simulink model "chase_1"  (R2017b)
settings: Solver=VariableStepAuto  StartTime=0.0  StopTime=400  FixedStep=0.0000001  RelTol=1e-3
values from neighbouring files (symbols this model uses):
  Cwy1 = 0.0074    [Parameters (2).m]    (also in Parameters.m)
  Cwy2 = 0.0527    [Parameters (2).m]    (also in Parameters.m)
  Cx = 52.92    [Parameters (2).m]    (also in Parameters.m)
  Jyy = 0.78    [Parameters (2).m]    (also in Parameters.m)
  k1_k = 0.3    [Parameters (2).m]    (also in Parameters.m)
  k2_k = 0.16732    [Parameters (2).m]    (also in Parameters.m)
  k2_m = 2.19    [Parameters (2).m]    (also in Parameters.m)
  K_thruster = 2.89    [Parameters (2).m]    (also in Parameters.m)
  kc = 57.2958    [Parameters (2).m]    (also in Parameters.m)
  L = 1.760    (= 1.76)    [Parameters (2).m]    (also in Parameters.m)
  lambda11 = 0.6    [Parameters (2).m]    (also in Parameters.m)
  lambda55 = 0.9    [Parameters (2).m]    (also in Parameters.m)
  m = 24.7    [Parameters (2).m]    (also in Parameters.m)
  Rmin = 0.4    [Parameters (2).m]    (also in Parameters.m)
  T_thruster = 0.1    [Parameters (2).m]    (also in Parameters.m)
libraries: simulink x5, simulink_extras x1
settings Model: Creator=Eugene  LastModifiedBy=Eugene
settings DebuggingCC: ParameterOverflowMsg=warning
settings HardwareCC: ProdHWDeviceType=AMD->x86-64 (Windows64)

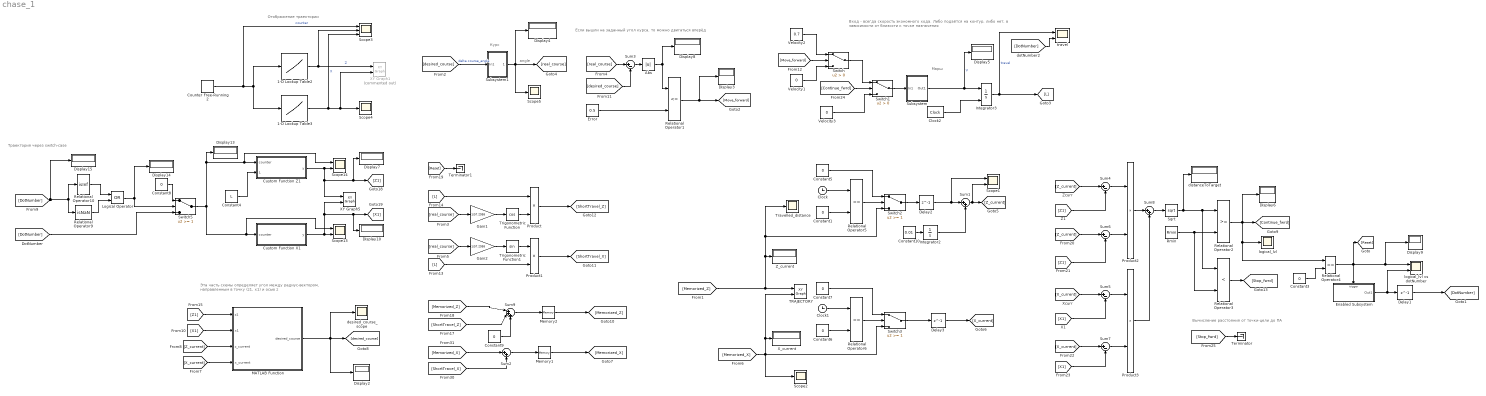
== system chase_1 ==
  note: Вход - всегда скорость экономного хода. Либо подаётся на контур, либо нет, в зависимости от близости к точке назначения
  note: Марш
  note: angle
  note: Курс
  note: Отображение траектории
  note: Вычисление расстояния от точки-цели до ПА
  note: Если вышли на заданный угол курса, то можно двигаться вперёд
  note: Траектория через switch-case
  note: Эта часть схемы определяет угол между радиус-вектором, направленным в точку (z1, x1) и осью z
  1-D Lookup Table2 : Lookup_n-D  NumberOfTableDimensions=1  BreakpointsForDimension1=[0:7]  BreakpointsForDimension1FirstPoint=0  BreakpointsForDimension1DataTypeStr=uint8  Table=[0,0,L,L,2*L,2*L,3*L, 3*L]  TableDataTypeStr=double  InterpMethod=Flat  ExtrapMethod=Cubic spline  RemoveProtectionInput=on  InternalRulePriority=Speed  OutDataTypeStr=double  RndMeth=Zero  InputSameDT=on
  1-D Lookup Table3 : Lookup_n-D  NumberOfTableDimensions=1  BreakpointsForDimension1=[0:7]  BreakpointsForDimension1DataTypeStr=int16  Table=[0,25,25,0,0,25,25,0]  TableDataTypeStr=double  InterpMethod=Flat  RemoveProtectionInput=on  InternalRulePriority=Speed  OutDataTypeStr=double  RndMeth=Zero  InputSameDT=on
  Abs : Abs
  Clock : Clock
  Clock1 : Clock
  Clock2 : simulink_extras/Flip Flops/Clock  period=0.05
  Constant{1,3,5..9} (7 alike) : Constant  Value=0
  Constant10 : Constant  Value=0.01
  Constant4 : Constant  Value=L
  Counter Free-Running2 : simulink/Sources/Counter Free-Running  NumBits=3  tsamp=1
  Custom Function X1 : MATLAB Function  TreatAsAtomicUnit=on
  Custom Function Z1 : MATLAB Function  TreatAsAtomicUnit=on
  Delay1 : Delay  DelayLength=1  SampleTime=0.05
  Delay2 : Delay  DelayLength=1  SampleTime=0.05
  Delay3 : Delay  DelayLength=1  SampleTime=0.05
  Display{2..10,13..15} (12 alike) : Display
  Enabled Subsystem : Subsystem  TreatAsAtomicUnit=on
  Error : Constant  Value=0.5
  Gain1 : Gain  Gain=1/57.2958
  Gain2 : Gain  Gain=1/57.2958
  Integrator2 : Integrator
  Integrator3 : Integrator  ExternalReset=rising
  Logical Operator : Logic  Operator=OR  AllPortsSameDT=off  OutDataTypeStr=boolean
  MATLAB Function : MATLAB Function  TreatAsAtomicUnit=on
  Memory1 : Memory
  Memory2 : Memory
  Product{,1..3} (4 alike) : Product
  Relational Operator1 : RelationalOperator  Operator=<=  OutDataTypeStr=boolean  RndMeth=Simplest
  Relational Operator10 : RelationalOperator  Operator=isInf  OutDataTypeStr=boolean  RndMeth=Simplest
  Relational Operator2 : RelationalOperator  OutDataTypeStr=boolean  RndMeth=Simplest
  Relational Operator3 : RelationalOperator  Operator=<  OutDataTypeStr=boolean  RndMeth=Simplest
  Relational Operator4 : RelationalOperator  Operator===  OutDataTypeStr=boolean  RndMeth=Simplest
  Relational Operator5 : RelationalOperator  Operator===  OutDataTypeStr=boolean  RndMeth=Simplest
  Relational Operator6 : RelationalOperator  Operator===  OutDataTypeStr=boolean  RndMeth=Simplest
  Relational Operator9 : RelationalOperator  Operator=isNaN  OutDataTypeStr=boolean  RndMeth=Simplest
  Rmin : Constant  Value=Rmin
  Scope1 : Scope  NumInputPorts=2
  Scope13 : Scope  NumInputPorts=2
  Scope14 : Scope  NumInputPorts=2
  Scope2 : Scope
  Scope3 : Scope  NumInputPorts=3
  Scope4 : Scope
  Scope5 : Scope
  Sqrt : Sqrt  SaturateOnIntegerOverflow=on
  Subsystem : Subsystem
  Subsystem1 : Subsystem
  Sum1 : Sum  Inputs=|++
  Sum2 : Sum  Inputs=|++
  Sum{3..7} (5 alike) : Sum  Inputs=|+-
  Sum8 : Sum  Inputs=|++
  Sum9 : Sum  Inputs=|+++
  Switch : Switch  Criteria=u2 > Threshold
  Switch1 : Switch  Criteria=u2 > Threshold
  Switch2 : Switch  Threshold=1
  Switch3 : Switch  Threshold=1
  Switch5 : Switch  Threshold=1
  TRAJECTORY : simulink/Sinks/XY Graph  xmin=-1  xmax=10  ymin=-5  ymax=30  st=-1
  Terminator : Terminator
  Terminator1 : Terminator
  Travelled_distance : Scope
  Trigonometric Function : Trigonometry  Operator=cos
  Trigonometric Function1 : Trigonometry
  Velocity1 : Constant  Value=0
  Velocity2 : Constant  Value=0.7
  Velocity3 : Constant  Value=0
  XY Graph1 : simulink/Sinks/XY Graph  Commented=on  xmin=-10  xmax=20  ymin=-10  ymax=30  st=-1
  XY Graph5 : simulink/Sinks/XY Graph  xmin=-1  xmax=10  ymin=-10  ymax=30  st=-1
  X_current : Display
  Z_current : Display
  desired_course_scope : Scope
  distanceToTarget : Display
  logical_lvl : Scope
  logical_lvl vs dotNumber : Scope  NumInputPorts=2
  travel : Scope  NumInputPorts=2
  wires:
  1-D Lookup Table3/1 -> Scope4/1, XY Graph1/2, Scope3/3  "X"
  1-D Lookup Table2/1 -> XY Graph1/1, Scope3/2  "Z"
  Counter Free-Running2/1 -> Scope3/1, 1-D Lookup Table2/1, 1-D Lookup Table3/1  "counter"
  Subsystem/1(Out1) -> Display5/1, Integrator3/1  "V"
  [desired_course] -> Subsystem1/1(In1)  "delta course_angle"
  Subsystem1/1(Out1) -> Display4/1, Scope5/1, [real_course]
  Trigonometric Function/1 -> Product/2
  [real_course] -> Gain1/1
  [real_course] -> Gain2/1
  Trigonometric Function1/1 -> Product1/1
  Integrator3/1 -> [L], travel/1  "travel"
  [real_course] -> Sum3/1
  [desired_course] -> Sum3/2
  Velocity2/1 -> Switch/1
  Velocity1/1 -> Switch/3
  Sum3/1 -> Abs/1
  Error/1 -> Relational Operator1/2
  Relational Operator1/1 -> [Move_forward], Display3/1
  [Move_forward] -> Switch/2
  [L] -> Product1/2
  [L] -> Product/1
  Gain1/1 -> Trigonometric Function/1
  Gain2/1 -> Trigonometric Function1/1
  [Z_current] -> Sum4/1
  [Z1] -> Sum4/2
  [X_current] -> Sum5/1
  [X1] -> Sum5/2
  [Z1] -> Sum6/2
  [Z_current] -> Sum6/1
  Sum4/1 -> Product2/1
  Sum6/1 -> Product2/2
  Sum5/1 -> Product3/1
  Sum7/1 -> Product3/2
  [X1] -> Sum7/2
  [X_current] -> Sum7/1
  Product2/1 -> Sum8/1
  Product3/1 -> Sum8/2
  Sum8/1 -> Sqrt/1
  Sqrt/1 -> Relational Operator2/1, Relational Operator3/1, distanceToTarget/1
  Rmin/1 -> Relational Operator2/2, Relational Operator3/2
  Relational Operator3/1 -> [Stop_fwrd]
  [Continue_fwrd] -> Switch1/2
  Switch/1 -> Switch1/1
  Switch1/1 -> Subsystem/1(In1)
  Velocity3/1 -> Switch1/3
  [Stop_fwrd] -> Terminator/1
  Relational Operator2/1 -> Display6/1, Relational Operator4/1, logical_lvl/1, [Continue_fwrd]
  Constant3/1 -> Relational Operator4/2
  Enabled Subsystem/1(Out1) -> Delay1/1, logical_lvl vs dotNumber/2
  Custom Function X1/1(y) -> Display10/1, [X1], XY Graph5/2, Scope13/2
  Custom Function Z1/1(y) -> Scope14/2, Display7/1, [Z1], XY Graph5/1
  Constant4/1 -> Custom Function Z1/2(L)
  Relational Operator4/1 -> [Reset], Enabled Subsystem/Trigger, logical_lvl vs dotNumber/1, Display9/1
  Switch5/1 -> Display13/1, Scope14/1, Custom Function Z1/1(counter), Scope13/1, Custom Function X1/1(counter)
  Delay1/1 -> [DotNumber]
  Clock2/1 -> Integrator3/2
  [DotNumber] -> travel/2
  Clock/1 -> Relational Operator5/1
  Constant1/1 -> Relational Operator5/2
  Relational Operator5/1 -> Switch2/2
  Constant5/1 -> Switch2/1
  Switch2/1 -> Delay2/1
  Constant7/1 -> Switch3/1
  Relational Operator6/1 -> Switch3/2
  Constant6/1 -> Relational Operator6/2
  Clock1/1 -> Relational Operator6/1
  [Memorized_X] -> Switch3/3, Scope2/1, TRAJECTORY/2, X_current/1
  Switch3/1 -> Delay3/1
  [DotNumber] -> Switch5/3
  Relational Operator10/1 -> Logical Operator/1
  [DotNumber] -> Display15/1, Relational Operator9/1, Relational Operator10/1
  Relational Operator9/1 -> Logical Operator/2
  Constant8/1 -> Switch5/1
  Logical Operator/1 -> Switch5/2, Display14/1
  Delay3/1 -> [X_current]
  Product1/1 -> [ShortTravel_X]
  [Reset] -> Terminator1/1
  Product/1 -> [ShortTravel_Z]
  [X1] -> MATLAB Function/2(x1)
  [Z_current] -> MATLAB Function/3(z_current)
  [X_current] -> MATLAB Function/4(x_current)
  MATLAB Function/1(desired_course) -> [desired_course], Display2/1, desired_course_scope/1
  [Z1] -> MATLAB Function/1(z1)
  [Memorized_X] -> Sum2/1
  Sum2/1 -> Memory1/1
  Memory1/1 -> [Memorized_X]
  [ShortTravel_X] -> Sum2/2
  Abs/1 -> Relational Operator1/1, Display8/1
  [ShortTravel_Z] -> Sum9/2
  Memory2/1 -> [Memorized_Z]
  Sum9/1 -> Memory2/1
  [Memorized_Z] -> Sum9/1
  Constant9/1 -> Sum9/3
  [Memorized_Z] -> Switch2/3, Travelled_distance/1, Z_current/1, TRAJECTORY/1
  Integrator2/1 -> Sum1/2
  Constant10/1 -> Integrator2/1
  Sum1/1 -> Scope1/2, [Z_current]
  Delay2/1 -> Scope1/1, Sum1/1

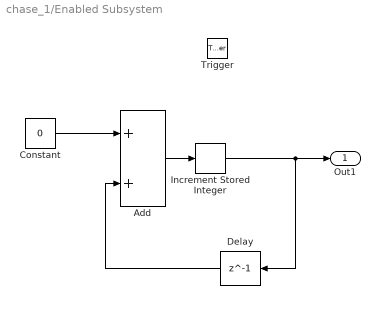
== system chase_1/Enabled Subsystem ==
  Trigger : TriggerPort  VariantControl=Variant  PortDimensions=1
  Add : Sum
  Constant : Constant  Value=0
  Delay : Delay  DelayLength=1  InitialCondition=0
  Increment Stored Integer : simulink/Additional Math & Discrete/Additional Math: Increment - Decrement/Increment Stored Integer
      settings: SourceProductName=Simulink
  Out1 : Outport
  wires:
  Constant/1 -> Add/1
  Delay/1 -> Add/2
  Add/1 -> Increment Stored Integer/1
  Increment Stored Integer/1 -> Delay/1, Out1/1

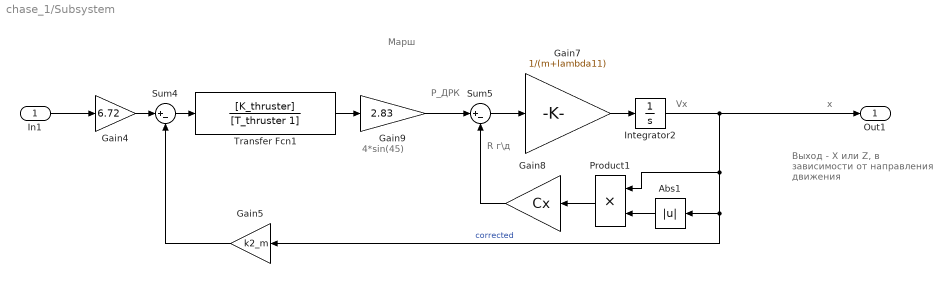
== system chase_1/Subsystem ==
  note: Выход - X или Z, в зависимости от направления движения
  note: 4*sin(45)
  note: R г\д
  note: x
  note: Vx
  note: P_ДРК
  note: Марш
  In1 : Inport
  Abs1 : Abs
  Gain4 : Gain  Gain=6.72
  Gain5 : Gain  Gain=k2_m
  Gain7 : Gain  Gain=1/(m+lambda11)
  Gain8 : Gain  Gain=Cx
  Gain9 : Gain  Gain=2.83
  Integrator2 : Integrator
  Product1 : Product
  Sum4 : Sum  Inputs=|+-
  Sum5 : Sum  Inputs=|+-
  Transfer Fcn1 : TransferFcn  Numerator=[K_thruster]  Denominator=[T_thruster 1]
  Out1 : Outport
  wires:
  In1/1 -> Gain4/1
  Product1/1 -> Gain8/1
  Gain7/1 -> Integrator2/1
  Gain8/1 -> Sum5/2
  Integrator2/1 -> Out1/1, Gain5/1, Abs1/1, Product1/1  "corrected"
  Transfer Fcn1/1 -> Gain9/1
  Gain4/1 -> Sum4/1
  Sum4/1 -> Transfer Fcn1/1
  Sum5/1 -> Gain7/1
  Gain9/1 -> Sum5/1
  Gain5/1 -> Sum4/2
  Abs1/1 -> Product1/2

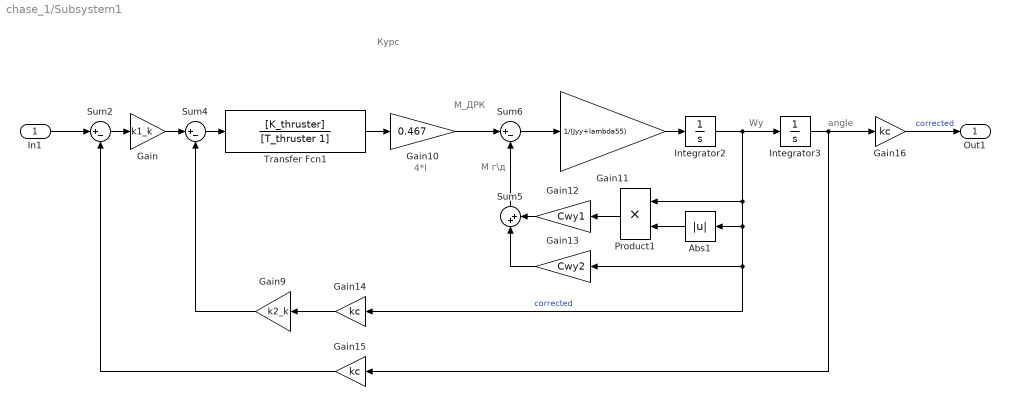
== system chase_1/Subsystem1 ==
  note: Курс
  note: Wy
  note: M_ДРК
  note: 4*l
  note: angle
  note: M г\д
  In1 : Inport
  Abs1 : Abs
  Gain : Gain  Gain=k1_k
  Gain10 : Gain  Gain=0.467
  Gain11 : Gain  Gain=1/(Jyy+lambda55)
  Gain12 : Gain  Gain=Cwy1
  Gain13 : Gain  Gain=Cwy2
  Gain14 : Gain  Gain=kc
  Gain15 : Gain  Gain=kc
  Gain16 : Gain  Gain=kc
  Gain9 : Gain  Gain=k2_k
  Integrator2 : Integrator
  Integrator3 : Integrator
  Product1 : Product
  Sum2 : Sum  Inputs=|+-
  Sum4 : Sum  Inputs=|+-
  Sum5 : Sum  Inputs=|++
  Sum6 : Sum  Inputs=|+-
  Transfer Fcn1 : TransferFcn  Numerator=[K_thruster]  Denominator=[T_thruster 1]
  Out1 : Outport
  wires:
  Gain12/1 -> Sum5/2
  Gain10/1 -> Sum6/1
  Product1/1 -> Gain12/1
  Gain11/1 -> Integrator2/1
  Gain9/1 -> Sum4/2
  Gain/1 -> Sum4/1
  Transfer Fcn1/1 -> Gain10/1
  Sum6/1 -> Gain11/1
  Gain14/1 -> Gain9/1
  Gain15/1 -> Sum2/2
  Gain13/1 -> Sum5/1
  Abs1/1 -> Product1/2
  Sum5/1 -> Sum6/2
  Integrator2/1 -> Gain14/1, Gain13/1, Abs1/1, Product1/1, Integrator3/1  "corrected"
  Sum2/1 -> Gain/1
  Integrator3/1 -> Gain16/1, Gain15/1
  Sum4/1 -> Transfer Fcn1/1
  In1/1 -> Sum2/1
  Gain16/1 -> Out1/1  "corrected"

== matlab function chase_1/Custom Function X1 ==
  data: counter input; y output
function y = fcn(counter)

%L = 1.76;

switch counter
    case 1
      y = 25;
    case 2
      y = 0;
    case 3
      y = 0;
    case 4
      y = 25;
    case 5
      y = 25;
    case 6
      y = 0;
    case 7
      y = 0;
    case 8
      y = 25;    
    case 9
      y = 25;
   otherwise
      y = 25;
end

== matlab function chase_1/Custom Function Z1 ==
  data: counter input; y output; L input
function y = fcn( counter, L)

%L = 1.76;

switch counter
    case 1
      y = L;
    case 2
      y = L;
    case 3
      y = 2*L;
    case 4
      y = 2*L;
    case 5
      y = 3*L;
    case 6
      y = 3*L;
    case 7
      y = 4*L;
    case 8
      y = 4*L;      
    case 9
      y = 5*L;      
   otherwise
      y = 0;
end

== matlab function chase_1/MATLAB Function ==
  data: z1 input; x1 input; z_current input; desired_course output; x_current input
function desired_course = fcn(z1, x1, z_current, x_current)

if z1 < z_current
    desired_course = 180 - 57.2958*atan((x1-x_current)/(abs(z1-z_current)));
else
    desired_course = 57.2958*atan((x1-x_current)/((z1-z_current)));
end
